simulink model "Simulaciones"  (R2020a)
settings: Solver=VariableStepAuto  StartTime=0.0  StopTime=5  RelTol=1e-3
undefined symbols (not defined in the file or in its folder): A, B, C, cdty, ceroanu, cnty, D1, dcont, denominador, denres, E, F, ganancia, gananciaanu, gananciares, Kd, KE, Ki, kih, Kiservo, Kp, N1, ncont, numanu, numerador, numres, Q0, Q1, Q2, S0, T, tiempo, tm, Ts, ts
settings Model: Creator=Usuario  LastModifiedBy=ladg1
settings DataIOCC: ReturnWorkspaceOutputs=off
settings DebuggingCC: ArithmeticOperatorsInVariantConditions=warning
settings SFSimCC: SimUseLocalCustomCode=off  CustomCodeUndefinedFunction=UseInterfaceOnly
settings RTWCC: RTWUseLocalCustomCode=off

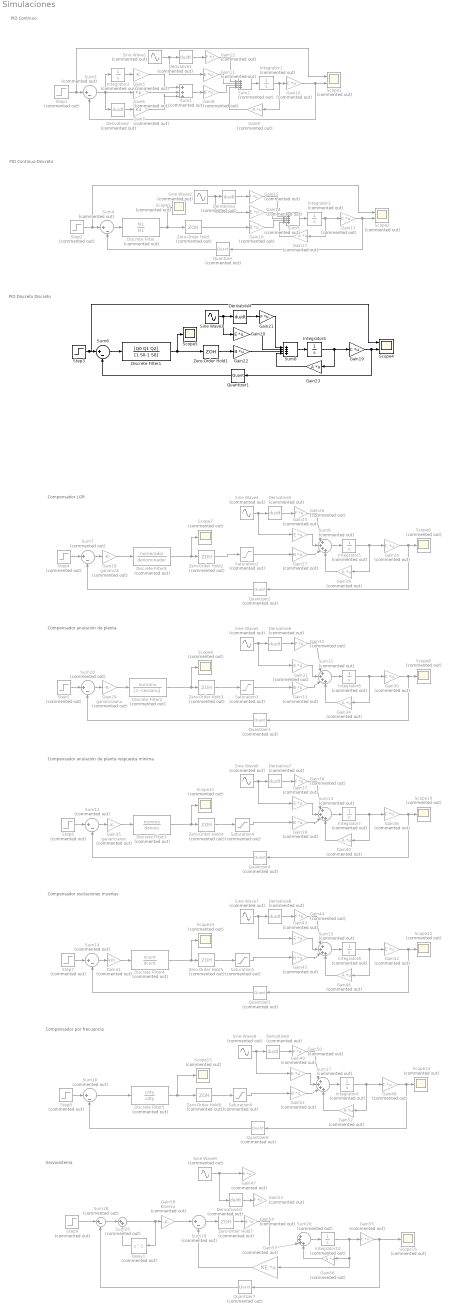
== system Simulaciones ==
  note: PID Discreto Discreto
  note: PID Continuo-Discreto
  note: PID Continuo
  note: Compensador LGR
  note: Compensador anulación de planta
  note: Compensador anulación de planta respuesta mínima
  note: Compensador oscilaciones muertas
  note: Compensador por frecuencia
  note: Servosistema
  Delay1 : Delay  Commented=on  DelayLength=1  SampleTime=Ts
  Derivative{1..3,5..10} (9 alike) : Derivative  Commented=on
  Derivative4 : Derivative
  Discrete Filter : DiscreteFilter  Commented=on  Numerator=N1  Denominator=D1  SampleTime=ts
  Discrete Filter1 : DiscreteFilter  Numerator=[Q0 Q1 Q2]  Denominator=[1 S0-1 S0]  SampleTime=tm
  Discrete Filter2 : DiscreteFilter  Commented=on  Numerator=numanu  Denominator=[1 -ceroanu]  SampleTime=tm
  Discrete Filter3 : DiscreteFilter  Commented=on  Numerator=numres  Denominator=denres  SampleTime=tm
  Discrete Filter4 : DiscreteFilter  Commented=on  Numerator=ncont  Denominator=dcont  SampleTime=tiempo
  Discrete Filter5 : DiscreteFilter  Commented=on  Numerator=cnty  Denominator=cdty  SampleTime=T
  Discrete Filter8 : DiscreteFilter  Commented=on  Numerator=numerador  Denominator=denominador  SampleTime=T
  Gain{10,13,24,30,36,42,48,55} (8 alike) : Gain  Commented=on  Gain=C  Multiplication=Matrix(K*u)
  Gain{11,14,25,31,37,43,47,49} (8 alike) : Gain  Commented=on  Gain=E  Multiplication=Matrix(K*u)
  Gain{12,15,26,32,38,44,50,53} (8 alike) : Gain  Commented=on  Gain=F  Multiplication=Matrix(K*u)
  Gain{8,16,27,33,39,45,51,54} (8 alike) : Gain  Commented=on  Gain=B  Multiplication=Matrix(K*u)
  Gain{9,17,28,34,40,46,52,56} (8 alike) : Gain  Commented=on  Gain=A  Multiplication=Matrix(K*u)
  Gain18 : Gain  Commented=on  Gain=ganancia
  Gain19 : Gain  Gain=C  Multiplication=Matrix(K*u)
  Gain20 : Gain  Gain=E  Multiplication=Matrix(K*u)
  Gain21 : Gain  Gain=F  Multiplication=Matrix(K*u)
  Gain22 : Gain  Gain=B  Multiplication=Matrix(K*u)
  Gain23 : Gain  Gain=A  Multiplication=Matrix(K*u)
  Gain29 : Gain  Commented=on  Gain=gananciaanu
  Gain35 : Gain  Commented=on  Gain=gananciares
  Gain41 : Gain  Commented=on  Gain=kih
  Gain5 : Gain  Commented=on  Gain=Ki
  Gain57 : Gain  Commented=on  Gain=KE  Multiplication=Matrix(K*u) (u vector)
  Gain58 : Gain  Commented=on  Gain=Kiservo
  Gain6 : Gain  Commented=on  Gain=Kp
  Gain7 : Gain  Commented=on  Gain=Kd
  Integrator{1,3,5..10} (8 alike) : Integrator  Commented=on  InitialCondition=-1
  Integrator2 : Integrator  Commented=on
  Integrator4 : Integrator  InitialCondition=-1
  Quantizer{,2..6} (6 alike) : Quantizer  Commented=on  QuantizationInterval=5/1048
  Quantizer1 : Quantizer  QuantizationInterval=5/1048
  Quantizer7 : Quantizer  Commented=on  QuantizationInterval=805.6640e-06
  Saturation{2..5} (4 alike) : Saturate  Commented=on  UpperLimit=100  LowerLimit=-100
  Saturation6 : Saturate  Commented=on  UpperLimit=30000  LowerLimit=-30000
  Scope1 : Scope  Commented=on  NumInputPorts=2
  Scope{3,6..16} (12 alike) : Scope  Commented=on
  Scope2 : Scope  Commented=on  NumInputPorts=2
  Scope4 : Scope  NumInputPorts=2
  Scope5 : Scope
  Sine Wave{1..2,4..9} (8 alike) : Sin  Commented=on  Amplitude=0.5  Frequency=pi/4  SampleTime=0
  Sine Wave3 : Sin  Amplitude=0.5  Frequency=pi/4  SampleTime=0
  Step1 : Step  Commented=on  Time=0  SampleTime=0
  Step2 : Step  Commented=on  Time=0  SampleTime=0
  Step3 : Step  Time=0  SampleTime=0
  Step{4..9} (6 alike) : Step  Commented=on  Time=0  After=0  SampleTime=0
  Sum1 : Sum  Commented=on  Inputs=|+++
  Sum{3..4,7,10,12,14,16,18..19} (9 alike) : Sum  Commented=on  Inputs=|+-
  Sum{2,5,9,11,13,15,17,20} (8 alike) : Sum  Commented=on  Inputs=|++++
  Sum25 : Sum  Commented=on  Inputs=|++
  Sum6 : Sum  Inputs=|+-
  Sum8 : Sum  Inputs=|++++
  Zero-Order Hold : ZeroOrderHold  Commented=on  SampleTime=ts
  Zero-Order Hold1 : ZeroOrderHold  SampleTime=tm
  Zero-Order Hold2 : ZeroOrderHold  Commented=on  SampleTime=T
  Zero-Order Hold3 : ZeroOrderHold  Commented=on  SampleTime=tm
  Zero-Order Hold4 : ZeroOrderHold  Commented=on  SampleTime=tm
  Zero-Order Hold5 : ZeroOrderHold  Commented=on  SampleTime=tiempo
  Zero-Order Hold6 : ZeroOrderHold  Commented=on  SampleTime=T
  Zero-Order Hold7 : ZeroOrderHold  Commented=on  SampleTime=Ts
  wires:
  Gain5/1 -> Sum1/1
  Gain6/1 -> Sum1/2
  Gain7/1 -> Sum1/3
  Integrator1/1 -> Gain9/1, Gain10/1
  Gain8/1 -> Sum2/3
  Derivative1/1 -> Gain12/1
  Sum2/1 -> Integrator1/1
  Sum1/1 -> Gain8/1
  Gain9/1 -> Sum2/4
  Sine Wave1/1 -> Gain11/1, Derivative1/1
  Gain10/1 -> Sum3/2, Scope1/2
  Sum3/1 -> Derivative2/1, Gain6/1, Integrator2/1
  Integrator2/1 -> Gain5/1
  Derivative2/1 -> Gain7/1
  Discrete Filter/1 -> Scope3/1, Zero-Order Hold/1
  Sum4/1 -> Discrete Filter/1
  Quantizer/1 -> Sum4/2
  Sine Wave2/1 -> Derivative3/1, Gain14/1
  Gain17/1 -> Sum5/4
  Zero-Order Hold/1 -> Gain16/1
  Sum5/1 -> Integrator3/1
  Derivative3/1 -> Gain15/1
  Gain16/1 -> Sum5/3
  Integrator3/1 -> Gain13/1, Gain17/1
  Gain13/1 -> Scope2/2, Quantizer/1
  Gain19/1 -> Scope4/2, Quantizer1/1
  Sum6/1 -> Discrete Filter1/1
  Sum7/1 -> Gain18/1
  Step4/1 -> Sum7/1
  Gain18/1 -> Discrete Filter8/1
  Integrator4/1 -> Gain23/1, Gain19/1
  Sine Wave3/1 -> Derivative4/1, Gain20/1
  Gain23/1 -> Sum8/4
  Gain22/1 -> Sum8/3
  Derivative4/1 -> Gain21/1
  Quantizer1/1 -> Sum6/2
  Sum8/1 -> Integrator4/1
  Saturation2/1 -> Gain27/1
  Zero-Order Hold2/1 -> Saturation2/1
  Derivative5/1 -> Gain26/1
  Sum9/1 -> Integrator5/1
  Quantizer2/1 -> Sum7/2
  Gain27/1 -> Sum9/3
  Gain28/1 -> Sum9/4
  Gain24/1 -> Scope6/1, Quantizer2/1
  Integrator5/1 -> Gain24/1, Gain28/1
  Discrete Filter8/1 -> Scope7/1, Zero-Order Hold2/1
  Sine Wave4/1 -> Derivative5/1, Gain25/1
  Sum10/1 -> Gain29/1
  Step5/1 -> Sum10/1
  Sine Wave5/1 -> Derivative6/1, Gain31/1
  Integrator6/1 -> Gain30/1, Gain34/1
  Gain34/1 -> Sum11/4
  Gain30/1 -> Scope8/1, Quantizer3/1
  Gain29/1 -> Discrete Filter2/1
  Gain33/1 -> Sum11/3
  Derivative6/1 -> Gain32/1
  Zero-Order Hold3/1 -> Saturation3/1
  Saturation3/1 -> Gain33/1
  Discrete Filter2/1 -> Scope9/1, Zero-Order Hold3/1
  Quantizer3/1 -> Sum10/2
  Sum11/1 -> Integrator6/1
  Discrete Filter1/1 -> Zero-Order Hold1/1, Scope5/1
  Quantizer4/1 -> Sum12/2
  Zero-Order Hold4/1 -> Saturation4/1
  Discrete Filter3/1 -> Scope11/1, Zero-Order Hold4/1
  Derivative7/1 -> Gain38/1
  Gain39/1 -> Sum13/3
  Gain36/1 -> Scope10/1, Quantizer4/1
  Gain40/1 -> Sum13/4
  Integrator7/1 -> Gain36/1, Gain40/1
  Gain35/1 -> Discrete Filter3/1
  Sine Wave6/1 -> Derivative7/1, Gain37/1
  Step6/1 -> Sum12/1
  Sum13/1 -> Integrator7/1
  Sum12/1 -> Gain35/1
  Saturation4/1 -> Gain39/1
  Gain42/1 -> Scope12/1, Quantizer5/1
  Derivative8/1 -> Gain44/1
  Quantizer5/1 -> Sum14/2
  Gain41/1 -> Discrete Filter4/1
  Zero-Order Hold5/1 -> Saturation5/1
  Saturation5/1 -> Gain45/1
  Sine Wave7/1 -> Derivative8/1, Gain43/1
  Gain45/1 -> Sum15/3
  Sum14/1 -> Gain41/1
  Integrator8/1 -> Gain42/1, Gain46/1
  Gain46/1 -> Sum15/4
  Discrete Filter4/1 -> Scope13/1, Zero-Order Hold5/1
  Sum15/1 -> Integrator8/1
  Step7/1 -> Sum14/1
  Sum17/1 -> Integrator9/1
  Integrator9/1 -> Gain48/1, Gain52/1
  Step8/1 -> Sum16/1
  Discrete Filter5/1 -> Scope15/1, Zero-Order Hold6/1
  Sum16/1 -> Discrete Filter5/1
  Saturation6/1 -> Gain51/1
  Zero-Order Hold6/1 -> Saturation6/1
  Sine Wave8/1 -> Derivative9/1, Gain49/1
  Gain48/1 -> Scope14/1, Quantizer6/1
  Gain52/1 -> Sum17/4
  Derivative9/1 -> Gain50/1
  Gain51/1 -> Sum17/3
  Quantizer6/1 -> Sum16/2
  Derivative10/1 -> Gain53/1
  Gain56/1 -> Sum20/4
  Delay1/1 -> Sum25/2
  Gain57/1 -> Sum19/2
  Sine Wave9/1 -> Derivative10/1, Gain47/1
  Quantizer7/1 -> Sum18/2
  Sum18/1 -> Sum25/1
  Step9/1 -> Sum18/1
  Gain55/1 -> Quantizer7/1, Scope16/1
  Gain58/1 -> Sum19/1
  Zero-Order Hold7/1 -> Gain54/1
  Sum19/1 -> Zero-Order Hold7/1
  Sum20/1 -> Integrator10/1
  Gain54/1 -> Sum20/3
  Integrator10/1 -> Gain57/1, Gain56/1, Gain55/1
  Sum25/1 -> Delay1/1, Gain58/1
  Gain38/1 -> Sum13/1
  Gain37/1 -> Sum13/2
  Gain25/1 -> Sum9/2
  Gain26/1 -> Sum9/1
  Gain21/1 -> Sum8/1
  Gain20/1 -> Sum8/2
  Gain12/1 -> Sum2/1
  Gain11/1 -> Sum2/2
  Gain32/1 -> Sum11/1
  Gain31/1 -> Sum11/2
  Gain49/1 -> Sum17/2
  Gain50/1 -> Sum17/1
  Gain44/1 -> Sum15/1
  Gain43/1 -> Sum15/2
  Gain15/1 -> Sum5/1
  Gain14/1 -> Sum5/2
  Step1/1 -> Sum3/1, Scope1/1
  Step2/1 -> Sum4/1, Scope2/1
  Zero-Order Hold1/1 -> Gain22/1
  Step3/1 -> Scope4/1, Sum6/1
